simulink model "test"  (R2020a)
settings: Solver=VariableStepAuto  StartTime=0.0  StopTime=10.0  RelTol=1e-3
values from neighbouring files (symbols this model uses):
  parameter = 4    [test.m]
settings Model: Creator=20200062  LastModifiedBy=20200062

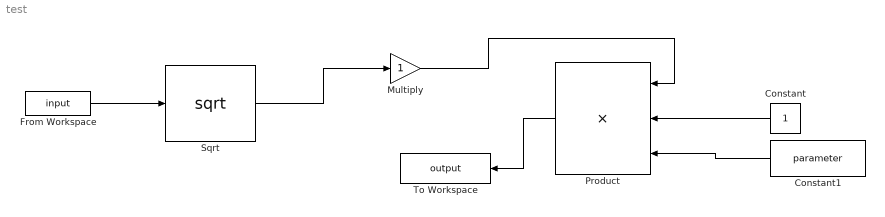
== system test ==
  Constant : Constant
  Constant1 : Constant  Value=parameter
  From Workspace : FromWorkspace  VariableName=input
  Multiply : Gain
  Product : Product  Inputs=3
  Sqrt : Sqrt  SaturateOnIntegerOverflow=on
  To Workspace : ToWorkspace  VariableName=output  SaveFormat=Timeseries  SampleTime=-1
  wires:
  Multiply/1 -> Product/1
  Sqrt/1 -> Multiply/1
  From Workspace/1 -> Sqrt/1
  Product/1 -> To Workspace/1
  Constant/1 -> Product/2
  Constant1/1 -> Product/3
